simulink model "A_Robot_2_0_m_5_V22_SI"  (R2025b)
settings: Solver=VariableStepAuto  StartTime=0.0  StopTime=150  RelTol=1e-3
model workspace (MAT data in the model file):
  Km = [1; 1]
values from neighbouring files (symbols this model uses):
  kcl = kil + 50    (= 75)    [A_init_0.m]    (also in A_init_0_v2.m; A_init_1_v2.m)
  kcr = kir + 50    (= 75)    [A_init_0.m]    (also in A_init_0_v2.m; A_init_1_v2.m)
  kil = 25    [A_init_0.m]    (also in A_init_0_v2.m; A_init_1_v2.m)
  kir = 25    [A_init_0.m]    (also in A_init_0_v2.m; A_init_1_v2.m)
  kpl = 5    [A_init_0.m]    (also in A_init_0_v2.m; A_init_1_v2.m)
  kpr = 5    [A_init_0.m]    (also in A_init_0_v2.m; A_init_1_v2.m)
  theta0 = theta_0_min + (theta_0_max - theta_0_min) * rand()    [A_init_0.m]    (also in A_init_0_v2.m; A_init_1_v2.m)
  theta_gsr = theta_gsr_min + (theta_gsr_max - theta_gsr_min) * rand()    [A_init_0.m]    (also in A_init_0_v2.m; A_init_1_v2.m)
  v_rand = v_rand_0 + (v_rand_max - v_rand_0) * rand()    [A_init_0.m]    (also in A_init_0_v2.m; A_init_1_v2.m)
  x0 = x_0_min + (x_0_max - x_0_min) * rand()    [A_init_0.m]    (also in A_init_0_v2.m; A_init_1_v2.m)
  x_gsr = x_gsr_min + (x_gsr_max - x_gsr_min) * rand()    [A_init_0.m]    (also in A_init_0_v2.m; A_init_1_v2.m)
  y0 = y_0_min + (y_0_max - y_0_min) * rand()    [A_init_0.m]    (also in A_init_0_v2.m; A_init_1_v2.m)
  y_gsr = y_gsr_min + (y_gsr_max - y_gsr_min) * rand()    [A_init_0.m]    (also in A_init_0_v2.m; A_init_1_v2.m)
undefined symbols (not defined in the file or in its folder): DiscIntNeverNeededParam
libraries: simulink x15, rllib x1
(part 3 of 3)

== matlab function A_Robot_2_0_m_5_V22_SI/MATLAB Function3 ==
  data: e_x input; done output; e_y input; e_theta input
function done = isDoneFcn(e_x, e_y, e_theta)
% isDoneFcn - określa, czy należy zakończyć epizod
% Warunki zakończenia:
%   - błąd pozycji > 0.5 m
%   - błąd orientacji > 90° (pi/2 rad)

% Progi graniczne
maxPosError = 2;               % [m]
maxThetaError = 2*pi;           % [rad] = 90 stopni

% Sprawdzenie warunków zakończenia
posViolation = norm([e_x, e_y]) > maxPosError;
thetaViolation = abs(e_theta) > maxThetaError;

% Epizod kończy się, gdy którykolwiek warunek jest spełniony
done = posViolation || thetaViolation;
end

== matlab function A_Robot_2_0_m_5_V22_SI/Model Robota 2.1/Model Dynamiki1/J^-1/MATLAB Function2 ==
  data: u input; Omega output; b input; r input
function Omega = predkosc_kotawa_kol(u, b, r)
% Oblicza prędkości kątowe kół napędowych Omega = [omega_P; omega_L]
% na podstawie wektora prędkości platformy u = [omega; v]
%
% Wejście:
%   u   - wektor prędkości platformy [omega; v] (rad/s, m/s)
%   b   - połowa rozstawu kół (odległość od osi do koła) [m]
%   r   - promień koła [m]
%
% Wyjście:
%   Omega - wektor prędkości kół [omega_P; omega_L] (rad/s)

% Macierz J^{-1} przekształcająca u -> Omega
J_1 = [b/r,1/r;
      -b/r,1/r];

% Obliczenie prędkości kątowych kół
Omega = J_1 * u;

end

== matlab function A_Robot_2_0_m_5_V22_SI/Model Robota 2.1/Model Dynamiki1/Km/MATLAB Function2 ==
  data: i_m input; Tm output; km input
function Tm = Km(i_m, km)
% Oblicza momenty napędowe Tm na podstawie prądów silników i_m
%
% Wejście:
%   i_m  – wektor prądów silników [i_mP; i_mL] (A)
%   km   – stała maszynowa silnika [N·m/A]
%
% Wyjście:
%   Tm   – wektor momentów napędowych [Tm_P; Tm_L] (N·m)

% Stała maszynowa jako macierz diagonalna
Km = km * eye(2);

% Obliczenie momentów napędowych
Tm = Km * i_m;

end

== matlab function A_Robot_2_0_m_5_V22_SI/MATLAB Function6 ==
  data: omega_dc input; omega_dsP output; ng input; omega_dsL output; omega_m_max input
function [omega_dsP, omega_dsL] = BSP(omega_dc, ng, omega_m_max)
% BSP - Blok Skalowania Prędkości
% Wejście:
%   omega_dcP, omega_dcL - zadane prędkości kół [rad/s]
%   r - promień koła [m]
%   b - połowa rozstawu kół [m]
%   ng - przełożenie przekładni
%   omega_m_max - maksymalna prędkość silnika [rad/s]
%
% Wyjście:
%   omega_dsP, omega_dsL - przeskalowane prędkości kół

    % Krok 1: Maksymalna prędkość koła
    omega_k_max = ng * omega_m_max;

    % Krok 2: Współczynnik skalujący (K1 z literatury)
    ks = max([1, abs(omega_dc(1))/omega_k_max, abs(omega_dc(2))/omega_k_max]);

    % Krok 3: Skalowanie zadanych prędkości kół (K2)
    omega_dsP = omega_dc(1) / ks;
    omega_dsL = omega_dc(2) / ks;
end

== matlab function A_Robot_2_0_m_5_V22_SI/MATLAB Function7 ==
  data: theta input; x input; y input; thetar input; xr input; yr input; u_dc output; vr input; wr input; k1 input; k2 input; k3 input
function u_dc  = ASP(theta, x, y, thetar, xr, yr, vr, wr, k1, k2, k3)


    % Obliczenie błędów pozycji w lokalnym układzie robota
    dx = xr - x;
    dy = yr - y;
    dtheta = wrapToPi(thetar - theta);

    % Przekształcenie błędów pozycji do układu robota
    e1 =  cos(theta) * dx + sin(theta) * dy;
    e2 = -sin(theta) * dx + cos(theta) * dy;
    e3 = dtheta;

    % Kinematyczna reguła sterowania
    v_c     = vr * cos(e3) + k1 * e1;
    omega_c = wr + k2 * vr * e2 + k3 * vr * sin(e3);

    u_dc=[omega_c;v_c];
end
